simulink subsystem "Motores2"  (R2024b)
settings: Solver=VariableStepAuto  StartTime=0.0  StopTime=10.0  RelTol=1e-3
libraries: arduinolib x6, simulink x2
settings Model: Creator=Laura  LastModifiedBy=Laura

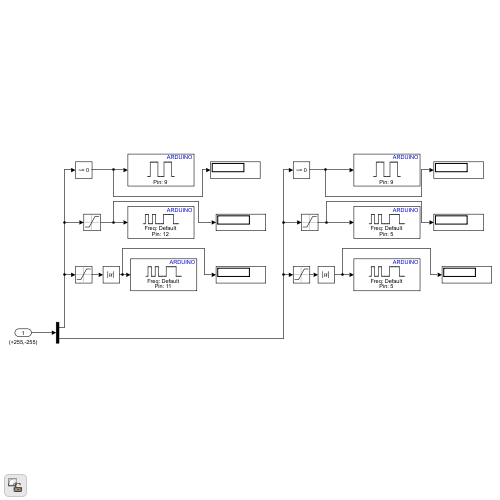
[thumbnail: Simulink's stored preview of the top-level diagram]
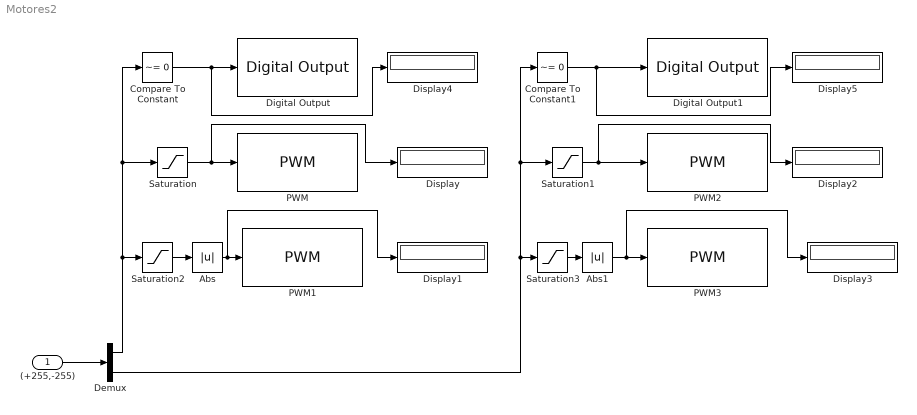
== system Motores2 ==
  (+255,-255) : Inport
  Abs : Abs  SaturateOnIntegerOverflow=off
  Abs1 : Abs  SaturateOnIntegerOverflow=off
  Compare To Constant : simulink/Logic and Bit Operations/Compare To Constant  relop=~=  const=0  OutDataTypeStr=boolean
  Compare To Constant1 : simulink/Logic and Bit Operations/Compare To Constant  relop=~=  const=0  OutDataTypeStr=boolean
  Demux : Demux  Outputs=2
  Digital Output : arduinolib/Digital Output  pinNumber=9  Direction=output  blockPlatform=arduino
  Digital Output1 : arduinolib/Digital Output  pinNumber=9  Direction=output  blockPlatform=arduino
  Display{,1..5} (6 alike) : Display
  PWM : arduinolib/PWM  pinNumber=12  frequencyType=Default  desiredFrequency=490.2  achievableFrequency=490.2
  PWM1 : arduinolib/PWM  pinNumber=11  frequencyType=Default  desiredFrequency=490.2  achievableFrequency=490.2
  PWM2 : arduinolib/PWM  pinNumber=5  frequencyType=Default  desiredFrequency=490.2  achievableFrequency=490.2
  PWM3 : arduinolib/PWM  pinNumber=5  frequencyType=Default  desiredFrequency=490.2  achievableFrequency=490.2
  Saturation : Saturate  UpperLimit=255  LowerLimit=0
  Saturation1 : Saturate  UpperLimit=255  LowerLimit=0
  Saturation2 : Saturate  UpperLimit=-1  LowerLimit=-255
  Saturation3 : Saturate  UpperLimit=-1  LowerLimit=-255
  wires:
  Compare To Constant/1 -> Display4/1, Digital Output/1
  Compare To Constant1/1 -> Display5/1, Digital Output1/1
  Demux/1 -> Saturation2/1, Saturation/1, Compare To Constant/1
  Demux/2 -> Saturation3/1, Saturation1/1, Compare To Constant1/1
  (+255,-255)/1 -> Demux/1
  Saturation/1 -> Display/1, PWM/1
  Saturation1/1 -> Display2/1, PWM2/1
  Saturation2/1 -> Abs/1
  Abs/1 -> Display1/1, PWM1/1
  Saturation3/1 -> Abs1/1
  Abs1/1 -> Display3/1, PWM3/1
